simulink model "sep_19"  (R2023a)
settings: Solver=FixedStepAuto  StartTime=0.0  StopTime=350  FixedStep=0.0001  RelTol=1e-3
settings Model: Creator=20808  LastModifiedBy=20808

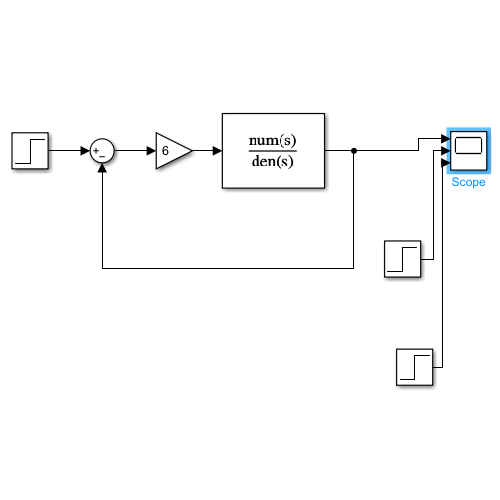
[thumbnail: Simulink's stored preview of the top-level diagram]
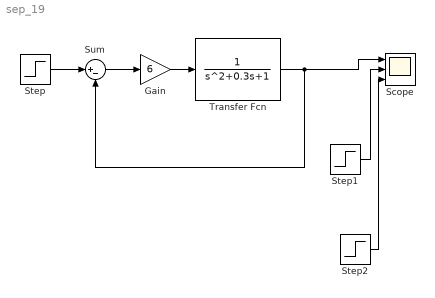
== system sep_19 ==
  Gain : Gain  Gain=6
  Scope : Scope  NumInputPorts=3
  Step : Step  Time=0  SampleTime=0
  Step1 : Step  Time=0  After=1.005  SampleTime=0
  Step2 : Step  Time=0  After=0.995  SampleTime=0
  Sum : Sum  Inputs=|+-
  Transfer Fcn : TransferFcn  Denominator=[1 0.3 1]
  wires:
  Transfer Fcn/1 -> Scope/1, Sum/2
  Step1/1 -> Scope/2
  Step2/1 -> Scope/3
  Step/1 -> Sum/1
  Gain/1 -> Transfer Fcn/1
  Sum/1 -> Gain/1
